simulink model "SImulink_model_solar_dryer"  (R2024b)
settings: Solver=VariableStepAuto  StartTime=0.0  StopTime=10.0  RelTol=1e-3
settings Model: Creator=chall  LastModifiedBy=chall

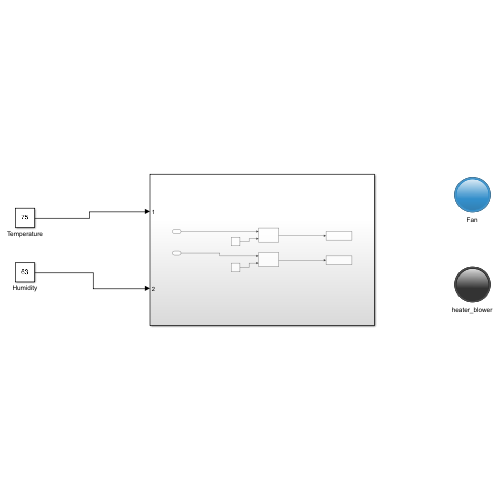
[thumbnail: Simulink's stored preview of the top-level diagram]
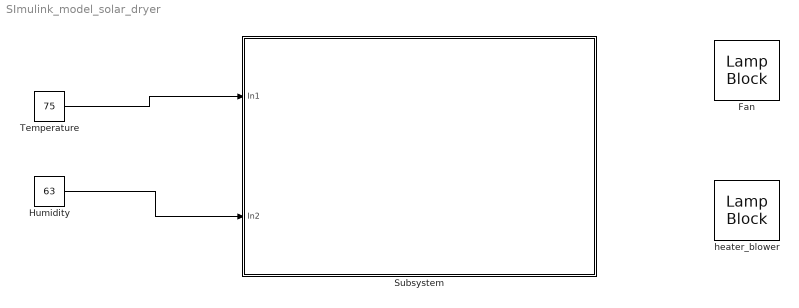
== system SImulink_model_solar_dryer ==
  Fan : LampBlock  LabelPosition=Hide
  Humidity : Constant  Value=63
  Subsystem : Subsystem
  Temperature : Constant  Value=75
  heater_blower : LampBlock  LabelPosition=Hide
  wires:
  Temperature/1 -> Subsystem/1(In1)
  Humidity/1 -> Subsystem/2(In2)

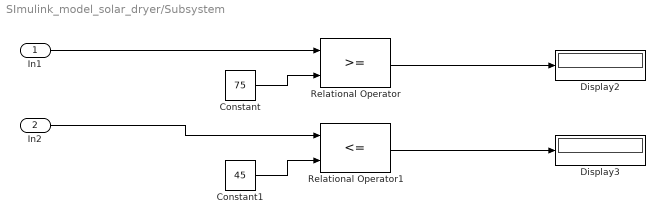
== system SImulink_model_solar_dryer/Subsystem ==
  In1 : Inport
  In2 : Inport  Port=2
  Constant : Constant  Value=75
  Constant1 : Constant  Value=45
  Display2 : Display
  Display3 : Display
  Relational Operator : RelationalOperator  OutDataTypeStr=boolean  RndMeth=Simplest  InputSameDT=off
  Relational Operator1 : RelationalOperator  Operator=<=  OutDataTypeStr=boolean  RndMeth=Simplest  InputSameDT=off
  wires:
  In1/1 -> Relational Operator/1
  Relational Operator/1 -> Display2/1
  Constant1/1 -> Relational Operator1/2
  Relational Operator1/1 -> Display3/1
  Constant/1 -> Relational Operator/2
  In2/1 -> Relational Operator1/1
